simulink model "robotarm_A2_breach"  (R2018b)
settings: Solver=FixedStepAuto  StartTime=0.0  StopTime=tspan(end)  RelTol=1e-3  AbsTol=1e-6
undefined symbols (not defined in the file): options
libraries: neural x132, simulink x2
(part 4 of 6)

== system robotarm_A2_breach/NN/Layer 3/Delays 1 ==
  "p{3}" : Inport  PortDimensions=30
      mask Display: e = 0.06;c1 = [120 230 180]/255;c2 = ([120 230 180]+0)/(256+128);c3 = ([120 230 180]+128)/(256+128);patch([0 1 1 0],[0 0 1 1],c1);patch([0 1 1 1-e 1-e 0+e],[0 0 1 1-e 0+e 0+e],c2);patch([0 0 1 1-e 0+e 0+e],[0 1 1 1-e 1-e 0+e],c3);plot([0 1 1 0 0],[0 0 1 1 0]);
  mux : Mux  Inputs=1
      mask Display: e = 0.06;c1 = [120 150 230]/255;c2 = ([120 150 230]+0)/383;c3 = ([120 150 230]+128)/383;patch([0 1 1 0],[0 0 1 1],c1);patch([0 1 1 1-e 1-e 0+e],[0 0 1 1-e 0+e 0+e],c2);patch([0 0 1 1-e 0+e 0+e],[0 1 1 1-e 1-e 0+e],c3);plot([0 1 1 0 0],[0 0 1 1 0]);disp('Mux')
  "pd{3,2}" : Outport
      mask Display: e = 0.06;c1 = [120 230 180]/255;c2 = ([120 230 180]+0)/(256+128);c3 = ([120 230 180]+128)/(256+128);patch([0 1 1 0],[0 0 1 1],c1);patch([0 1 1 1-e 1-e 0+e],[0 0 1 1-e 0+e 0+e],c2);patch([0 0 1 1-e 0+e 0+e],[0 1 1 1-e 1-e 0+e],c3);plot([0 1 1 0 0],[0 0 1 1 0]);
  wires:
  "p{3}"/1 -> mux/1
  mux/1 -> "pd{3,2}"/1

== system robotarm_A2_breach/NN/Layer 3/LW{3,2} ==
  "ad{3,2}" : Inport  PortDimensions=30
      mask Display: e = 0.06;c1 = [120 230 180]/255;c2 = ([120 230 180]+0)/(256+128);c3 = ([120 230 180]+128)/(256+128);patch([0 1 1 0],[0 0 1 1],c1);patch([0 1 1 1-e 1-e 0+e],[0 0 1 1-e 0+e 0+e],c2);patch([0 0 1 1-e 0+e 0+e],[0 1 1 1-e 1-e 0+e],c3);plot([0 1 1 0 0],[0 0 1 1 0]);
  "IW{3,2}(1,:)'" : Constant  Value=[0.0612835242484911224547516894745058380067348480224609375;0.55401861205358493567274535962496884167194366455078125;-0.0309290079940963656690566807583309127949178218841552734375;0.0588484153819546218500136092188768088817596435546875;0.37185389163203641516020070412196218967437744140625;-0.08102638935974972034248509089593426324427127838134765625;-0.0160636941765267271531314463572925888001918792724609375;0.0141065889033629258964008812426982331089675426483154296875;0.093361899623724708963123930516303516924381256103515625;0.00928528364726113018823294709136462188325822353363037109375;0.01380683464663637859126676943333222880028188228607177734375;0.0120059251069379140097748148718892480246722698211669921875;0.2465228382685667185558742175999213941395282745361328125;0.289936215663593122027208437430090270936489105224609375;-0.2326784576660662906544274619591305963695049285888671875;-0.0444339979498476200792111967530217953026294708251953125;-0.52069617671258450197768752332194708287715911865234375;0.046310094473405470638649461534441797994077205657958984375;-0.0157586866225218717729728012955092708580195903778076171875;0.057788370293653475162631849570971098728477954864501953125;-0.041849453455607053820042295910752727650105953216552734375;-0.37515319116971579394004265850526280701160430908203125;0.01257613541710286657326900439102246309630572795867919921875;0.1998150780203487852926258483421406708657741546630859375;-0.216886981729346006719794104355969466269016265869140625;-0.1552099887166240310687470582706737332046031951904296875;-6.7795182034169758117543580500097277763416059315204620361328125e-06;0.040379623554425737863571299612885923124849796295166015625;-0.50160768795489329985315407611778937280178070068359375;0.57643069847345140832572951694601215422153472900390625]
      mask Display: e = 0.06;c1 = [120 150 230]/255;c2 = ([120 150 230]+0)/383;c3 = ([120 150 230]+128)/383;patch([0 1 1 0],[0 0 1 1],c1);patch([0 1 1 1-e 1-e 0+e],[0 0 1 1-e 0+e 0+e],c2);patch([0 0 1 1-e 0+e 0+e],[0 1 1 1-e 1-e 0+e],c3);plot([0 1 1 0 0],[0 0 1 1 0]);disp('weights');
  Mux : Mux  Inputs=1
      mask Display: e = 0.06;c1 = [120 150 230]/255;c2 = ([120 150 230]+0)/383;c3 = ([120 150 230]+128)/383;patch([0 1 1 0],[0 0 1 1],c1);patch([0 1 1 1-e 1-e 0+e],[0 0 1 1-e 0+e 0+e],c2);patch([0 0 1 1-e 0+e 0+e],[0 1 1 1-e 1-e 0+e],c3);plot([0 1 1 0 0],[0 0 1 1 0]);disp('Mux');
  dotprod1 : neural/Weight Functions/dotprod
  "lz{3,2}" : Outport
      mask Display: e = 0.06;c1 = [120 230 180]/255;c2 = ([120 230 180]+0)/(256+128);c3 = ([120 230 180]+128)/(256+128);patch([0 1 1 0],[0 0 1 1],c1);patch([0 1 1 1-e 1-e 0+e],[0 0 1 1-e 0+e 0+e],c2);patch([0 0 1 1-e 0+e 0+e],[0 1 1 1-e 1-e 0+e],c3);plot([0 1 1 0 0],[0 0 1 1 0]);
  wires:
  "IW{3,2}(1,:)'"/1 -> dotprod1/1
  "ad{3,2}"/1 -> dotprod1/2
  dotprod1/1 -> Mux/1
  Mux/1 -> "lz{3,2}"/1

== system robotarm_A2_breach/NN_cex_1/Layer 1/Delays 1 ==
  "p{1}" : Inport  PortDimensions=10
      mask Display: e = 0.06;c1 = [120 230 180]/255;c2 = ([120 230 180]+0)/(256+128);c3 = ([120 230 180]+128)/(256+128);patch([0 1 1 0],[0 0 1 1],c1);patch([0 1 1 1-e 1-e 0+e],[0 0 1 1-e 0+e 0+e],c2);patch([0 0 1 1-e 0+e 0+e],[0 1 1 1-e 1-e 0+e],c3);plot([0 1 1 0 0],[0 0 1 1 0]);
  mux : Mux  Inputs=1
      mask Display: e = 0.06;c1 = [120 150 230]/255;c2 = ([120 150 230]+0)/383;c3 = ([120 150 230]+128)/383;patch([0 1 1 0],[0 0 1 1],c1);patch([0 1 1 1-e 1-e 0+e],[0 0 1 1-e 0+e 0+e],c2);patch([0 0 1 1-e 0+e 0+e],[0 1 1 1-e 1-e 0+e],c3);plot([0 1 1 0 0],[0 0 1 1 0]);disp('Mux')
  "pd{1,1}" : Outport
      mask Display: e = 0.06;c1 = [120 230 180]/255;c2 = ([120 230 180]+0)/(256+128);c3 = ([120 230 180]+128)/(256+128);patch([0 1 1 0],[0 0 1 1],c1);patch([0 1 1 1-e 1-e 0+e],[0 0 1 1-e 0+e 0+e],c2);patch([0 0 1 1-e 0+e 0+e],[0 1 1 1-e 1-e 0+e],c3);plot([0 1 1 0 0],[0 0 1 1 0]);
  wires:
  "p{1}"/1 -> mux/1
  mux/1 -> "pd{1,1}"/1

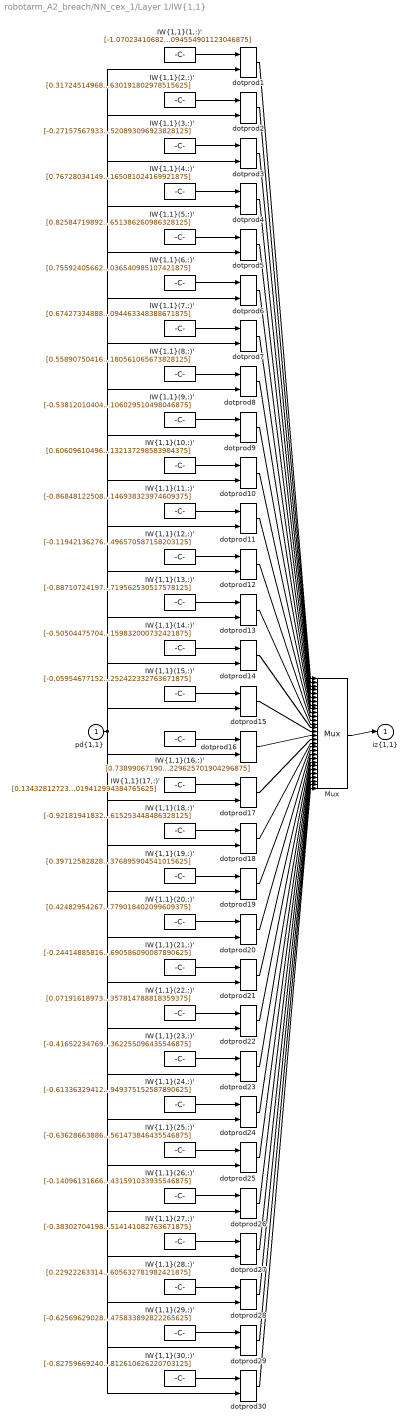
== system robotarm_A2_breach/NN_cex_1/Layer 1/IW{1,1} ==
  "pd{1,1}" : Inport  PortDimensions=10
      mask Display: e = 0.06;c1 = [120 230 180]/255;c2 = ([120 230 180]+0)/(256+128);c3 = ([120 230 180]+128)/(256+128);patch([0 1 1 0],[0 0 1 1],c1);patch([0 1 1 1-e 1-e 0+e],[0 0 1 1-e 0+e 0+e],c2);patch([0 0 1 1-e 0+e 0+e],[0 1 1 1-e 1-e 0+e],c3);plot([0 1 1 0 0],[0 0 1 1 0]);
  "IW{1,1}(1,:)'" : Constant  Value=[-1.0702341068269236590282389443018473684787750244140625;-0.429136666934705035547636953197070397436618804931640625;-0.2643524669662393744573591902735643088817596435546875;-0.625004900318298250994075715425424277782440185546875;-0.8824456949316503706626235725707374513149261474609375;0.4083420833766615576365666129277087748050689697265625;-0.71200655701400716868221252298098988831043243408203125;-0.020905446514137178415371209894146886654198169708251953125;-0.1369270488505061056372369421296752989292144775390625;0.122515490039902086305545481081935577094554901123046875]
      mask Display: e = 0.06;c1 = [120 150 230]/255;c2 = ([120 150 230]+0)/383;c3 = ([120 150 230]+128)/383;patch([0 1 1 0],[0 0 1 1],c1);patch([0 1 1 1-e 1-e 0+e],[0 0 1 1-e 0+e 0+e],c2);patch([0 0 1 1-e 0+e 0+e],[0 1 1 1-e 1-e 0+e],c3);plot([0 1 1 0 0],[0 0 1 1 0]);disp('Weights');
  "IW{1,1}(10,:)'" : Constant  Value=[0.606096104962364545798436665791086852550506591796875;0.47600429883855144286286531496443785727024078369140625;0.55968923618874466541228684945963323116302490234375;-0.35367784161168136503050618557608686387538909912109375;-0.386942654117144291259222654844052158296108245849609375;-0.404596446105812412863400595597340725362300872802734375;0.76258899534525703689524789297138340771198272705078125;-0.89448893238682469775113759169471450150012969970703125;0.044060317281896514696182265424795332364737987518310546875;0.06527498170639166319428881024578004144132137298583984375]
      mask Display: e = 0.06;c1 = [120 150 230]/255;c2 = ([120 150 230]+0)/383;c3 = ([120 150 230]+128)/383;patch([0 1 1 0],[0 0 1 1],c1);patch([0 1 1 1-e 1-e 0+e],[0 0 1 1-e 0+e 0+e],c2);patch([0 0 1 1-e 0+e 0+e],[0 1 1 1-e 1-e 0+e],c3);plot([0 1 1 0 0],[0 0 1 1 0]);disp('Weights');
  "IW{1,1}(11,:)'" : Constant  Value=[-0.868481225086314534422626820742152631282806396484375;0.574366938918856373419430383364669978618621826171875;0.48581014030425961891523911617696285247802734375;-0.597890844506349328213445915025658905506134033203125;0.1276777768702727355876191950301290489733219146728515625;-1.0191648453984480937606349471025168895721435546875;-0.18178946502776793803235477753332816064357757568359375;-0.480534504324701072786041322615346871316432952880859375;0.84073664364318279051957460978883318603038787841796875;0.5364895751129414858127120169228874146938323974609375]
      mask Display: e = 0.06;c1 = [120 150 230]/255;c2 = ([120 150 230]+0)/383;c3 = ([120 150 230]+128)/383;patch([0 1 1 0],[0 0 1 1],c1);patch([0 1 1 1-e 1-e 0+e],[0 0 1 1-e 0+e 0+e],c2);patch([0 0 1 1-e 0+e 0+e],[0 1 1 1-e 1-e 0+e],c3);plot([0 1 1 0 0],[0 0 1 1 0]);disp('Weights');
  "IW{1,1}(12,:)'" : Constant  Value=[-0.1194213627673995359312897335257730446755886077880859375;-0.77819285512311198171886417185305617749691009521484375;0.6971419994382268559007798103266395628452301025390625;0.255631948433803712905643124031485058367252349853515625;-0.67658981525328965034304928849451243877410888671875;1.1295921720586414860321156083955429494380950927734375;-0.829091418576481498092789479414932429790496826171875;0.331949112921899713857243341408320702612400054931640625;0.95089153391239167323334413595148362219333648681640625;1.2121869418178061739155282339197583496570587158203125]
      mask Display: e = 0.06;c1 = [120 150 230]/255;c2 = ([120 150 230]+0)/383;c3 = ([120 150 230]+128)/383;patch([0 1 1 0],[0 0 1 1],c1);patch([0 1 1 1-e 1-e 0+e],[0 0 1 1-e 0+e 0+e],c2);patch([0 0 1 1-e 0+e 0+e],[0 1 1 1-e 1-e 0+e],c3);plot([0 1 1 0 0],[0 0 1 1 0]);disp('Weights');
  "IW{1,1}(13,:)'" : Constant  Value=[-0.88710724197875390206746715193730778992176055908203125;0.7443291249174956991652152282767929136753082275390625;-0.7766695448863034645370362341054715216159820556640625;0.6560377192476438690249551655142568051815032958984375;0.1903690360253666724599241888427059166133403778076171875;-0.13900728286681951484382580019882880151271820068359375;0.2042442924484920430128198631791747175157070159912109375;-0.397701432840284530012553432243294082581996917724609375;0.40170295279101131402654800695017911493778228759765625;0.2223005438394709820659755905580823309719562530517578125]
      mask Display: e = 0.06;c1 = [120 150 230]/255;c2 = ([120 150 230]+0)/383;c3 = ([120 150 230]+128)/383;patch([0 1 1 0],[0 0 1 1],c1);patch([0 1 1 1-e 1-e 0+e],[0 0 1 1-e 0+e 0+e],c2);patch([0 0 1 1-e 0+e 0+e],[0 1 1 1-e 1-e 0+e],c3);plot([0 1 1 0 0],[0 0 1 1 0]);disp('Weights');
  "IW{1,1}(14,:)'" : Constant  Value=[-0.505044757043746184166366219869814813137054443359375;-0.64054944306781214091728315906948409974575042724609375;-0.48249039594317688628422047258936800062656402587890625;-0.2187822787071866670327580095545272342860698699951171875;0.05784663144858250005686528538717539049685001373291015625;-0.5355954538863070268916999339126050472259521484375;-0.1275687406131100487538532206599484197795391082763671875;-0.87970633518317697951971467773546464741230010986328125;0.63052476357508757676129107494489289820194244384765625;-0.8524120413610425384121072056586854159832000732421875]
      mask Display: e = 0.06;c1 = [120 150 230]/255;c2 = ([120 150 230]+0)/383;c3 = ([120 150 230]+128)/383;patch([0 1 1 0],[0 0 1 1],c1);patch([0 1 1 1-e 1-e 0+e],[0 0 1 1-e 0+e 0+e],c2);patch([0 0 1 1-e 0+e 0+e],[0 1 1 1-e 1-e 0+e],c3);plot([0 1 1 0 0],[0 0 1 1 0]);disp('Weights');
  "IW{1,1}(15,:)'" : Constant  Value=[-0.0595467715244530904072917110170237720012664794921875;0.51394639437917477575723523841588757932186126708984375;-0.2097622122006522482617896230294718407094478607177734375;-0.479944235182659995064824443034012801945209503173828125;1.188802688797679696364184565027244389057159423828125;0.441158950532180182957375791374943219125270843505859375;-0.68205384793610190907742207855335436761379241943359375;0.243789964149355942168995170504786074161529541015625;-0.83837980184352389745328082426567561924457550048828125;-0.59381907631233843414264583771000616252422332763671875]
      mask Display: e = 0.06;c1 = [120 150 230]/255;c2 = ([120 150 230]+0)/383;c3 = ([120 150 230]+128)/383;patch([0 1 1 0],[0 0 1 1],c1);patch([0 1 1 1-e 1-e 0+e],[0 0 1 1-e 0+e 0+e],c2);patch([0 0 1 1-e 0+e 0+e],[0 1 1 1-e 1-e 0+e],c3);plot([0 1 1 0 0],[0 0 1 1 0]);disp('Weights');
  "IW{1,1}(16,:)'" : Constant  Value=[0.73899067190857803399950398670625872910022735595703125;-0.318935108048426896321103640730143524706363677978515625;0.78790778130619887331675954555976204574108123779296875;-0.325386417923637372151546287568635307252407073974609375;0.54282934625056833422007684930576942861080169677734375;-0.57864627066384277664923274642205797135829925537109375;-0.039075083981605092386946154192628455348312854766845703125;0.77214547540941469438990907292463816702365875244140625;0.81030144108731383401078574024722911417484283447265625;-0.365158741097107775175345523166470229625701904296875]
      mask Display: e = 0.06;c1 = [120 150 230]/255;c2 = ([120 150 230]+0)/383;c3 = ([120 150 230]+128)/383;patch([0 1 1 0],[0 0 1 1],c1);patch([0 1 1 1-e 1-e 0+e],[0 0 1 1-e 0+e 0+e],c2);patch([0 0 1 1-e 0+e 0+e],[0 1 1 1-e 1-e 0+e],c3);plot([0 1 1 0 0],[0 0 1 1 0]);disp('Weights');
  "IW{1,1}(17,:)'" : Constant  Value=[0.134328127235650851556414409060380421578884124755859375;0.344243463874768007570992267574183642864227294921875;0.0270789085382987550210120986093897954560816287994384765625;1.08739690118722709399889936321415007114410400390625;0.93017418921626326966389797235024161636829376220703125;0.353239457851165894464173788946936838328838348388671875;0.387496438874461113233138576106284745037555694580078125;0.61943267756236430887639698994462378323078155517578125;-0.070521993643866076606485648881061933934688568115234375;-0.65473232388958158001202036757604219019412994384765625]
      mask Display: e = 0.06;c1 = [120 150 230]/255;c2 = ([120 150 230]+0)/383;c3 = ([120 150 230]+128)/383;patch([0 1 1 0],[0 0 1 1],c1);patch([0 1 1 1-e 1-e 0+e],[0 0 1 1-e 0+e 0+e],c2);patch([0 0 1 1-e 0+e 0+e],[0 1 1 1-e 1-e 0+e],c3);plot([0 1 1 0 0],[0 0 1 1 0]);disp('Weights');
  "IW{1,1}(18,:)'" : Constant  Value=[-0.92181941832154590255044013247243128716945648193359375;0.60393844708402910637090599266230128705501556396484375;-0.455977184568810034459573898857343010604381561279296875;0.80212877620000799794297563494183123111724853515625;-0.047491489147747534271815084139234386384487152099609375;0.81039293254306976610479296141420491039752960205078125;-0.95284720050586979578355339981499128043651580810546875;0.11637158261936685066384455922161578200757503509521484375;0.299979759085471087143304202982108108699321746826171875;-0.352458494814660128202632449756492860615253448486328125]
      mask Display: e = 0.06;c1 = [120 150 230]/255;c2 = ([120 150 230]+0)/383;c3 = ([120 150 230]+128)/383;patch([0 1 1 0],[0 0 1 1],c1);patch([0 1 1 1-e 1-e 0+e],[0 0 1 1-e 0+e 0+e],c2);patch([0 0 1 1-e 0+e 0+e],[0 1 1 1-e 1-e 0+e],c3);plot([0 1 1 0 0],[0 0 1 1 0]);disp('Weights');
  "IW{1,1}(19,:)'" : Constant  Value=[0.397125828288026505585861514191492460668087005615234375;-1.073941230155850856675670002005062997341156005859375;0.50267383535256071613872563830227591097354888916015625;-0.487548977472428368695744893557275645434856414794921875;-0.439408986445312788049477603635750710964202880859375;-0.04336928758741422085254413332222611643373966217041015625;-0.94940255590337796487432342473766766488552093505859375;0.136945129813424271159050249480060301721096038818359375;0.0143810557676019752648688410090471734292805194854736328125;-0.80499842494032292083971924512297846376895904541015625]
      mask Display: e = 0.06;c1 = [120 150 230]/255;c2 = ([120 150 230]+0)/383;c3 = ([120 150 230]+128)/383;patch([0 1 1 0],[0 0 1 1],c1);patch([0 1 1 1-e 1-e 0+e],[0 0 1 1-e 0+e 0+e],c2);patch([0 0 1 1-e 0+e 0+e],[0 1 1 1-e 1-e 0+e],c3);plot([0 1 1 0 0],[0 0 1 1 0]);disp('Weights');
  "IW{1,1}(2,:)'" : Constant  Value=[0.31724514968994810271141204793821088969707489013671875;0.053901704580535829414156268057922716252505779266357421875;-0.89308984743340946721446016454137861728668212890625;0.5066985683601530343622698637773282825946807861328125;-0.805641429036569878263662758399732410907745361328125;0.75489638673323400386294679265120066702365875244140625;-0.32645743368310864429560069766012020409107208251953125;0.81363995271355860072759469403536058962345123291015625;-0.572761549458138841117715855943970382213592529296875;-0.174957972377838277822093004942871630191802978515625]
      mask Display: e = 0.06;c1 = [120 150 230]/255;c2 = ([120 150 230]+0)/383;c3 = ([120 150 230]+128)/383;patch([0 1 1 0],[0 0 1 1],c1);patch([0 1 1 1-e 1-e 0+e],[0 0 1 1-e 0+e 0+e],c2);patch([0 0 1 1-e 0+e 0+e],[0 1 1 1-e 1-e 0+e],c3);plot([0 1 1 0 0],[0 0 1 1 0]);disp('Weights');
  "IW{1,1}(20,:)'" : Constant  Value=[0.4248295426769634897112837279564701020717620849609375;-0.698589515854909137715367251075804233551025390625;-0.51207957663037306783593294312595389783382415771484375;-0.434033759553325904079201791319064795970916748046875;-0.57289499322343362397447208422818221151828765869140625;-0.956669489742406842225364016485400497913360595703125;-0.1411078779893085999308510736227617599070072174072265625;0.5921261100055115189633170302840881049633026123046875;-0.438179607713289509529630549877765588462352752685546875;0.2366247377450834965539883114615804515779018402099609375]
      mask Display: e = 0.06;c1 = [120 150 230]/255;c2 = ([120 150 230]+0)/383;c3 = ([120 150 230]+128)/383;patch([0 1 1 0],[0 0 1 1],c1);patch([0 1 1 1-e 1-e 0+e],[0 0 1 1-e 0+e 0+e],c2);patch([0 0 1 1-e 0+e 0+e],[0 1 1 1-e 1-e 0+e],c3);plot([0 1 1 0 0],[0 0 1 1 0]);disp('Weights');
  "IW{1,1}(21,:)'" : Constant  Value=[-0.2441488581620429865193244722831877879798412322998046875;1.0906900279345472792869031763984821736812591552734375;-0.836079316872020417150679350015707314014434814453125;0.194568724325025199650696094977320171892642974853515625;-0.3575090898695825192277197857038117945194244384765625;-0.23986124457636670559423919257824309170246124267578125;0.89241596363539754666049930165172554552555084228515625;0.30315433800865687619108257422340102493762969970703125;-0.69896753043077775036095999894314445555210113525390625;0.447550700116873034772879691445268690586090087890625]
      mask Display: e = 0.06;c1 = [120 150 230]/255;c2 = ([120 150 230]+0)/383;c3 = ([120 150 230]+128)/383;patch([0 1 1 0],[0 0 1 1],c1);patch([0 1 1 1-e 1-e 0+e],[0 0 1 1-e 0+e 0+e],c2);patch([0 0 1 1-e 0+e 0+e],[0 1 1 1-e 1-e 0+e],c3);plot([0 1 1 0 0],[0 0 1 1 0]);disp('Weights');
  "IW{1,1}(22,:)'" : Constant  Value=[0.07191618973229686739845334386700415052473545074462890625;-0.1783347113074600087667676007185946218669414520263671875;-0.79705447543285956601977204627473838627338409423828125;0.38208697743551478520629416379961185157299041748046875;-0.434634390661599534499970332035445608198642730712890625;1.0959968122559100578428115113638341426849365234375;-0.2057036542755317498620826199839939363300800323486328125;0.4717110549411216435800042745540849864482879638671875;0.34772738202242603477998272865079343318939208984375;-0.67527564422144903399924942277721129357814788818359375]
      mask Display: e = 0.06;c1 = [120 150 230]/255;c2 = ([120 150 230]+0)/383;c3 = ([120 150 230]+128)/383;patch([0 1 1 0],[0 0 1 1],c1);patch([0 1 1 1-e 1-e 0+e],[0 0 1 1-e 0+e 0+e],c2);patch([0 0 1 1-e 0+e 0+e],[0 1 1 1-e 1-e 0+e],c3);plot([0 1 1 0 0],[0 0 1 1 0]);disp('Weights');
  "IW{1,1}(23,:)'" : Constant  Value=[-0.4165223476910318023413992705172859132289886474609375;0.1585156632944082211178482566538150422275066375732421875;0.9385971155881345229232692872756160795688629150390625;-0.68781285637631750518039552844129502773284912109375;-0.07559698228676466069675399239713442511856555938720703125;-0.56835921916896003924790647943154908716678619384765625;-0.7173276790399960578525906385038979351520538330078125;0.8642734118728061520897654190775938332080841064453125;-0.6652973933758534741400580969639122486114501953125;-0.0279961747111670648802128624765828135423362255096435546875]
      mask Display: e = 0.06;c1 = [120 150 230]/255;c2 = ([120 150 230]+0)/383;c3 = ([120 150 230]+128)/383;patch([0 1 1 0],[0 0 1 1],c1);patch([0 1 1 1-e 1-e 0+e],[0 0 1 1-e 0+e 0+e],c2);patch([0 0 1 1-e 0+e 0+e],[0 1 1 1-e 1-e 0+e],c3);plot([0 1 1 0 0],[0 0 1 1 0]);disp('Weights');
  "IW{1,1}(24,:)'" : Constant  Value=[-0.6133632941293176710217949221259914338588714599609375;1.4482686191216143090088053213548846542835235595703125;0.2495590181793570228041545533415046520531177520751953125;-0.271262462537200377266088935357402078807353973388671875;0.61406431548851447832504391044494695961475372314453125;-0.6517050058197231265921800513751804828643798828125;-0.8902317029364603673258216076646931469440460205078125;-0.02257125201677044612491584985036752186715602874755859375;-0.250293192032376321520814599352888762950897216796875;0.022676088013246921415433376978398882783949375152587890625]
      mask Display: e = 0.06;c1 = [120 150 230]/255;c2 = ([120 150 230]+0)/383;c3 = ([120 150 230]+128)/383;patch([0 1 1 0],[0 0 1 1],c1);patch([0 1 1 1-e 1-e 0+e],[0 0 1 1-e 0+e 0+e],c2);patch([0 0 1 1-e 0+e 0+e],[0 1 1 1-e 1-e 0+e],c3);plot([0 1 1 0 0],[0 0 1 1 0]);disp('Weights');
  "IW{1,1}(25,:)'" : Constant  Value=[-0.63628663886688097139909814359270967543125152587890625;0.7382589980125704443025824730284512042999267578125;0.023234489370555000409268586736288852989673614501953125;0.2560217799690722717542712416616268455982208251953125;-1.3069316061269777851094886500504799187183380126953125;0.02320568872151014538918190055483137257397174835205078125;0.52722279199295252194445993154658935964107513427734375;-0.373843584065578660169393288015271537005901336669921875;0.4753972732582363303066586013301275670528411865234375;0.07813696927503814559923256410911562852561473846435546875]
      mask Display: e = 0.06;c1 = [120 150 230]/255;c2 = ([120 150 230]+0)/383;c3 = ([120 150 230]+128)/383;patch([0 1 1 0],[0 0 1 1],c1);patch([0 1 1 1-e 1-e 0+e],[0 0 1 1-e 0+e 0+e],c2);patch([0 0 1 1-e 0+e 0+e],[0 1 1 1-e 1-e 0+e],c3);plot([0 1 1 0 0],[0 0 1 1 0]);disp('Weights');
  "IW{1,1}(26,:)'" : Constant  Value=[-0.14096131666791145153894149189000017940998077392578125;-0.3313433851921505635118592181243002414703369140625;-0.625230851216644456513904515304602682590484619140625;0.42600478489425686046132568662869744002819061279296875;0.6995294034281209771819476372911594808101654052734375;-0.29421230843110046659916179123683832585811614990234375;0.7583320558493766849750272740493528544902801513671875;-0.1046050124057833208279788550498778931796550750732421875;0.886966071100088182532772407284937798976898193359375;-0.8884478329492491166519130274537019431591033935546875]
      mask Display: e = 0.06;c1 = [120 150 230]/255;c2 = ([120 150 230]+0)/383;c3 = ([120 150 230]+128)/383;patch([0 1 1 0],[0 0 1 1],c1);patch([0 1 1 1-e 1-e 0+e],[0 0 1 1-e 0+e 0+e],c2);patch([0 0 1 1-e 0+e 0+e],[0 1 1 1-e 1-e 0+e],c3);plot([0 1 1 0 0],[0 0 1 1 0]);disp('Weights');
  "IW{1,1}(27,:)'" : Constant  Value=[-0.3830270419866217412874220826779492199420928955078125;0.84248017458946578006617755818297155201435089111328125;-0.8150440035837716035160838146111927926540374755859375;0.1584159392711783909124534375223447568714618682861328125;0.26381204178818162819908366145682521164417266845703125;-1.3183300267735920119349657397833652794361114501953125;0.88736245201829222484235515366890467703342437744140625;0.400267817919197799181318941919016651809215545654296875;0.2127421886728322608650643132932600565254688262939453125;-0.4113956660921302965761015002499334514141082763671875]
      mask Display: e = 0.06;c1 = [120 150 230]/255;c2 = ([120 150 230]+0)/383;c3 = ([120 150 230]+128)/383;patch([0 1 1 0],[0 0 1 1],c1);patch([0 1 1 1-e 1-e 0+e],[0 0 1 1-e 0+e 0+e],c2);patch([0 0 1 1-e 0+e 0+e],[0 1 1 1-e 1-e 0+e],c3);plot([0 1 1 0 0],[0 0 1 1 0]);disp('Weights');
  "IW{1,1}(28,:)'" : Constant  Value=[0.229222633142930565242068041698075830936431884765625;0.875781151993403117472780650132335722446441650390625;0.3580517592593508435783178356359712779521942138671875;-0.424759891657964738787001124364905990660190582275390625;0.862714476959423937074689092696644365787506103515625;0.05035102251195734679445337178549380041658878326416015625;0.33328571267431950087001268911990337073802947998046875;-0.59483987626800771675306123142945580184459686279296875;0.7758688061196290508547690478735603392124176025390625;0.463117263855785221693395214970223605632781982421875]
      mask Display: e = 0.06;c1 = [120 150 230]/255;c2 = ([120 150 230]+0)/383;c3 = ([120 150 230]+128)/383;patch([0 1 1 0],[0 0 1 1],c1);patch([0 1 1 1-e 1-e 0+e],[0 0 1 1-e 0+e 0+e],c2);patch([0 0 1 1-e 0+e 0+e],[0 1 1 1-e 1-e 0+e],c3);plot([0 1 1 0 0],[0 0 1 1 0]);disp('Weights');
  "IW{1,1}(29,:)'" : Constant  Value=[-0.62569629028702333783940048306249082088470458984375;0.8818350270248573874454223187058232724666595458984375;-0.257373906217436054788549881777726113796234130859375;-0.0628046437967268722513125567274983040988445281982421875;0.52359599739727002987166315506328828632831573486328125;-1.03417853367037881895384998642839491367340087890625;0.1358476420852212651624313366482965648174285888671875;0.4289884144587745584686899746884591877460479736328125;0.499903549717121198359137679290142841637134552001953125;-0.43922031492535273944355367348180152475833892822265625]
      mask Display: e = 0.06;c1 = [120 150 230]/255;c2 = ([120 150 230]+0)/383;c3 = ([120 150 230]+128)/383;patch([0 1 1 0],[0 0 1 1],c1);patch([0 1 1 1-e 1-e 0+e],[0 0 1 1-e 0+e 0+e],c2);patch([0 0 1 1-e 0+e 0+e],[0 1 1 1-e 1-e 0+e],c3);plot([0 1 1 0 0],[0 0 1 1 0]);disp('Weights');
  "IW{1,1}(3,:)'" : Constant  Value=[-0.27157567933646309388251438576844520866870880126953125;-0.7126343768502814146614809942548163235187530517578125;-0.74939698676090671369820483960211277008056640625;0.51749371875504757145591838707332499325275421142578125;0.10423103348294671111062825730186887085437774658203125;0.97480409491253727782833493620273657143115997314453125;-0.6284938839696219137209709515445865690708160400390625;0.89103197970491476720411583301029168069362640380859375;-0.59998828910454149454523076201439835131168365478515625;-0.2486797619840033224392072952468879520893096923828125]
      mask Display: e = 0.06;c1 = [120 150 230]/255;c2 = ([120 150 230]+0)/383;c3 = ([120 150 230]+128)/383;patch([0 1 1 0],[0 0 1 1],c1);patch([0 1 1 1-e 1-e 0+e],[0 0 1 1-e 0+e 0+e],c2);patch([0 0 1 1-e 0+e 0+e],[0 1 1 1-e 1-e 0+e],c3);plot([0 1 1 0 0],[0 0 1 1 0]);disp('Weights');
  "IW{1,1}(30,:)'" : Constant  Value=[-0.82759669240066424666935063214623369276523590087890625;-0.69259980019391764738401207068818621337413787841796875;-0.31378991321418470139548162478604353964328765869140625;0.885597945258245200506053151912055909633636474609375;0.46041529336223019353013796717277728021144866943359375;-0.077725831217165308739680540384142659604549407958984375;-0.79525883660562202148724963990389369428157806396484375;0.462328610603190248706795273392344824969768524169921875;-0.371187942647590418676628587490995414555072784423828125;0.2154875654783001692749166977591812610626220703125]
      mask Display: e = 0.06;c1 = [120 150 230]/255;c2 = ([120 150 230]+0)/383;c3 = ([120 150 230]+128)/383;patch([0 1 1 0],[0 0 1 1],c1);patch([0 1 1 1-e 1-e 0+e],[0 0 1 1-e 0+e 0+e],c2);patch([0 0 1 1-e 0+e 0+e],[0 1 1 1-e 1-e 0+e],c3);plot([0 1 1 0 0],[0 0 1 1 0]);disp('Weights');
  "IW{1,1}(4,:)'" : Constant  Value=[0.76728034149881896297529237926937639713287353515625;0.127483094780900307885218580850050784647464752197265625;0.9201298564872468777053882149630226194858551025390625;-0.227385232819694582673264449113048613071441650390625;0.1916046212127310022221848839762969873845577239990234375;0.531825462418062056002554527367465198040008544921875;-0.86846034924426607215508511217194609344005584716796875;0.2328950409211323069325061396739329211413860321044921875;0.4961021835192689355409356721793301403522491455078125;0.5957269264231548344667999117518775165081024169921875]
      mask Display: e = 0.06;c1 = [120 150 230]/255;c2 = ([120 150 230]+0)/383;c3 = ([120 150 230]+128)/383;patch([0 1 1 0],[0 0 1 1],c1);patch([0 1 1 1-e 1-e 0+e],[0 0 1 1-e 0+e 0+e],c2);patch([0 0 1 1-e 0+e 0+e],[0 1 1 1-e 1-e 0+e],c3);plot([0 1 1 0 0],[0 0 1 1 0]);disp('Weights');
  "IW{1,1}(5,:)'" : Constant  Value=[0.82584719892108260363983163188095204532146453857421875;-0.62527263456634718519211446619010530412197113037109375;0.07334159897852231269066436425418942235410213470458984375;-0.03691052496805451166306255572635564021766185760498046875;-0.0760550045288510556673600149224512279033660888671875;0.11891915159648747124521150908549316227436065673828125;0.769144020799244376718206694931723177433013916015625;-0.0331942018271159933195946223349892534315586090087890625;-0.21551264095972599843520356444059871137142181396484375;1.0243166979697235774438013322651386260986328125]
      mask Display: e = 0.06;c1 = [120 150 230]/255;c2 = ([120 150 230]+0)/383;c3 = ([120 150 230]+128)/383;patch([0 1 1 0],[0 0 1 1],c1);patch([0 1 1 1-e 1-e 0+e],[0 0 1 1-e 0+e 0+e],c2);patch([0 0 1 1-e 0+e 0+e],[0 1 1 1-e 1-e 0+e],c3);plot([0 1 1 0 0],[0 0 1 1 0]);disp('Weights');
  "IW{1,1}(6,:)'" : Constant  Value=[0.75592405662496819918061419230070896446704864501953125;0.77071666997196353054988549047266133129596710205078125;-0.97432636280755680058263124010409228503704071044921875;0.0538637780241819630333566237823106348514556884765625;-0.6455335776745272369225858710706233978271484375;1.0354771288624495806374170570052228868007659912109375;-0.61347735909790757080628509356756694614887237548828125;-0.556788356191117106419596893829293549060821533203125;-0.1538269614370491311650113175346632488071918487548828125;-0.2114579652654713093351546149278874509036540985107421875]
      mask Display: e = 0.06;c1 = [120 150 230]/255;c2 = ([120 150 230]+0)/383;c3 = ([120 150 230]+128)/383;patch([0 1 1 0],[0 0 1 1],c1);patch([0 1 1 1-e 1-e 0+e],[0 0 1 1-e 0+e 0+e],c2);patch([0 0 1 1-e 0+e 0+e],[0 1 1 1-e 1-e 0+e],c3);plot([0 1 1 0 0],[0 0 1 1 0]);disp('Weights');
  "IW{1,1}(7,:)'" : Constant  Value=[0.6742733488873657865525501620140857994556427001953125;-0.765981264248496440671942764311097562313079833984375;0.484131515779223808859654809566563926637172698974609375;0.534225617008788677964048474677838385105133056640625;-0.021428144658800808708409846303766244091093540191650390625;-0.5715061895560993310283492974122054874897003173828125;-0.63723018316298418728393926357966847717761993408203125;-0.01536985488226780445508712347191249136812984943389892578125;0.1090106235483598584590225755164283327758312225341796875;0.483663628504379772277133042734931223094463348388671875]
      mask Display: e = 0.06;c1 = [120 150 230]/255;c2 = ([120 150 230]+0)/383;c3 = ([120 150 230]+128)/383;patch([0 1 1 0],[0 0 1 1],c1);patch([0 1 1 1-e 1-e 0+e],[0 0 1 1-e 0+e 0+e],c2);patch([0 0 1 1-e 0+e 0+e],[0 1 1 1-e 1-e 0+e],c3);plot([0 1 1 0 0],[0 0 1 1 0]);disp('Weights');
  "IW{1,1}(8,:)'" : Constant  Value=[0.5589075041622637574079135447391308844089508056640625;-0.6910933115687918348868379325722344219684600830078125;-0.0694853618729556476996123137723770923912525177001953125;-0.1664297312980232701473681800052872858941555023193359375;-0.1812648065326095403460016086683026514947414398193359375;0.51827259240606926571359736044541932642459869384765625;-0.8741962245158096944663839167333208024501800537109375;0.42512105782948150789479768718592822551727294921875;0.52540100090166108603995098746963776648044586181640625;0.75192399924898822849428370318491943180561065673828125]
      mask Display: e = 0.06;c1 = [120 150 230]/255;c2 = ([120 150 230]+0)/383;c3 = ([120 150 230]+128)/383;patch([0 1 1 0],[0 0 1 1],c1);patch([0 1 1 1-e 1-e 0+e],[0 0 1 1-e 0+e 0+e],c2);patch([0 0 1 1-e 0+e 0+e],[0 1 1 1-e 1-e 0+e],c3);plot([0 1 1 0 0],[0 0 1 1 0]);disp('Weights');
  "IW{1,1}(9,:)'" : Constant  Value=[-0.5381201040443281957692533978843130171298980712890625;0.87066175699864623016566156366025097668170928955078125;-0.87975567905515894562284984203870408236980438232421875;-0.349977327794832426821614035361562855541706085205078125;0.6579708693633665728128789851325564086437225341796875;-0.1788772598580825323733023424210841767489910125732421875;-0.484773498860190665826763734003179706633090972900390625;0.381208719779995153231766380486078560352325439453125;-0.466309175065127867743086653717909939587116241455078125;0.12771998415035479279566743571194820106029510498046875]
      mask Display: e = 0.06;c1 = [120 150 230]/255;c2 = ([120 150 230]+0)/383;c3 = ([120 150 230]+128)/383;patch([0 1 1 0],[0 0 1 1],c1);patch([0 1 1 1-e 1-e 0+e],[0 0 1 1-e 0+e 0+e],c2);patch([0 0 1 1-e 0+e 0+e],[0 1 1 1-e 1-e 0+e],c3);plot([0 1 1 0 0],[0 0 1 1 0]);disp('Weights');
  Mux : Mux  Inputs=30
      mask Display: e = 0.06;c1 = [120 150 230]/255;c2 = ([120 150 230]+0)/383;c3 = ([120 150 230]+128)/383;patch([0 1 1 0],[0 0 1 1],c1);patch([0 1 1 1-e 1-e 0+e],[0 0 1 1-e 0+e 0+e],c2);patch([0 0 1 1-e 0+e 0+e],[0 1 1 1-e 1-e 0+e],c3);plot([0 1 1 0 0],[0 0 1 1 0]);disp('Mux');
  dotprod{1..30} (30 alike) : neural/Weight Functions/dotprod
  "iz{1,1}" : Outport
      mask Display: e = 0.06;c1 = [120 230 180]/255;c2 = ([120 230 180]+0)/(256+128);c3 = ([120 230 180]+128)/(256+128);patch([0 1 1 0],[0 0 1 1],c1);patch([0 1 1 1-e 1-e 0+e],[0 0 1 1-e 0+e 0+e],c2);patch([0 0 1 1-e 0+e 0+e],[0 1 1 1-e 1-e 0+e],c3);plot([0 1 1 0 0],[0 0 1 1 0]);
  wires:
  "IW{1,1}(1,:)'"/1 -> dotprod1/1
  "pd{1,1}"/1 -> dotprod1/2, dotprod2/2, dotprod3/2, dotprod4/2, dotprod5/2, dotprod6/2, dotprod7/2, dotprod8/2, dotprod9/2, dotprod10/2, dotprod11/2, dotprod12/2, dotprod13/2, dotprod14/2, dotprod15/2, dotprod16/2, dotprod17/2, dotprod18/2, dotprod19/2, dotprod20/2, dotprod21/2, dotprod22/2, dotprod23/2, dotprod24/2, dotprod25/2, dotprod26/2, dotprod27/2, dotprod28/2, dotprod29/2, dotprod30/2
  dotprod1/1 -> Mux/1
  "IW{1,1}(2,:)'"/1 -> dotprod2/1
  dotprod2/1 -> Mux/2
  "IW{1,1}(3,:)'"/1 -> dotprod3/1
  dotprod3/1 -> Mux/3
  "IW{1,1}(4,:)'"/1 -> dotprod4/1
  dotprod4/1 -> Mux/4
  "IW{1,1}(5,:)'"/1 -> dotprod5/1
  dotprod5/1 -> Mux/5
  "IW{1,1}(6,:)'"/1 -> dotprod6/1
  dotprod6/1 -> Mux/6
  "IW{1,1}(7,:)'"/1 -> dotprod7/1
  dotprod7/1 -> Mux/7
  "IW{1,1}(8,:)'"/1 -> dotprod8/1
  dotprod8/1 -> Mux/8
  "IW{1,1}(9,:)'"/1 -> dotprod9/1
  dotprod9/1 -> Mux/9
  "IW{1,1}(10,:)'"/1 -> dotprod10/1
  dotprod10/1 -> Mux/10
  "IW{1,1}(11,:)'"/1 -> dotprod11/1
  dotprod11/1 -> Mux/11
  "IW{1,1}(12,:)'"/1 -> dotprod12/1
  dotprod12/1 -> Mux/12
  "IW{1,1}(13,:)'"/1 -> dotprod13/1
  dotprod13/1 -> Mux/13
  "IW{1,1}(14,:)'"/1 -> dotprod14/1
  dotprod14/1 -> Mux/14
  "IW{1,1}(15,:)'"/1 -> dotprod15/1
  dotprod15/1 -> Mux/15
  "IW{1,1}(16,:)'"/1 -> dotprod16/1
  dotprod16/1 -> Mux/16
  "IW{1,1}(17,:)'"/1 -> dotprod17/1
  dotprod17/1 -> Mux/17
  "IW{1,1}(18,:)'"/1 -> dotprod18/1
  dotprod18/1 -> Mux/18
  "IW{1,1}(19,:)'"/1 -> dotprod19/1
  dotprod19/1 -> Mux/19
  "IW{1,1}(20,:)'"/1 -> dotprod20/1
  dotprod20/1 -> Mux/20
  "IW{1,1}(21,:)'"/1 -> dotprod21/1
  dotprod21/1 -> Mux/21
  "IW{1,1}(22,:)'"/1 -> dotprod22/1
  dotprod22/1 -> Mux/22
  "IW{1,1}(23,:)'"/1 -> dotprod23/1
  dotprod23/1 -> Mux/23
  "IW{1,1}(24,:)'"/1 -> dotprod24/1
  dotprod24/1 -> Mux/24
  "IW{1,1}(25,:)'"/1 -> dotprod25/1
  dotprod25/1 -> Mux/25
  "IW{1,1}(26,:)'"/1 -> dotprod26/1
  dotprod26/1 -> Mux/26
  "IW{1,1}(27,:)'"/1 -> dotprod27/1
  dotprod27/1 -> Mux/27
  "IW{1,1}(28,:)'"/1 -> dotprod28/1
  dotprod28/1 -> Mux/28
  "IW{1,1}(29,:)'"/1 -> dotprod29/1
  dotprod29/1 -> Mux/29
  "IW{1,1}(30,:)'"/1 -> dotprod30/1
  dotprod30/1 -> Mux/30
  Mux/1 -> "iz{1,1}"/1

== system robotarm_A2_breach/NN_cex_1/Layer 2/Delays 1 ==
  "p{2}" : Inport  PortDimensions=30
      mask Display: e = 0.06;c1 = [120 230 180]/255;c2 = ([120 230 180]+0)/(256+128);c3 = ([120 230 180]+128)/(256+128);patch([0 1 1 0],[0 0 1 1],c1);patch([0 1 1 1-e 1-e 0+e],[0 0 1 1-e 0+e 0+e],c2);patch([0 0 1 1-e 0+e 0+e],[0 1 1 1-e 1-e 0+e],c3);plot([0 1 1 0 0],[0 0 1 1 0]);
  mux : Mux  Inputs=1
      mask Display: e = 0.06;c1 = [120 150 230]/255;c2 = ([120 150 230]+0)/383;c3 = ([120 150 230]+128)/383;patch([0 1 1 0],[0 0 1 1],c1);patch([0 1 1 1-e 1-e 0+e],[0 0 1 1-e 0+e 0+e],c2);patch([0 0 1 1-e 0+e 0+e],[0 1 1 1-e 1-e 0+e],c3);plot([0 1 1 0 0],[0 0 1 1 0]);disp('Mux')
  "pd{2,1}" : Outport
      mask Display: e = 0.06;c1 = [120 230 180]/255;c2 = ([120 230 180]+0)/(256+128);c3 = ([120 230 180]+128)/(256+128);patch([0 1 1 0],[0 0 1 1],c1);patch([0 1 1 1-e 1-e 0+e],[0 0 1 1-e 0+e 0+e],c2);patch([0 0 1 1-e 0+e 0+e],[0 1 1 1-e 1-e 0+e],c3);plot([0 1 1 0 0],[0 0 1 1 0]);
  wires:
  "p{2}"/1 -> mux/1
  mux/1 -> "pd{2,1}"/1
